simulink library "HDL_ieee_8021513"  (R2024a)
settings: Solver=FixedStepDiscrete  StartTime=0.0  StopTime=10.0  RelTol=1e-3
undefined symbols (not defined in the file or in its folder): Add, axiWidth, channelCyclicPrefixLen, channelDataCarriers, channelEstReference, channelLUT, channelOFDMSamples, channelScramblerInit, decimatorDelay, decimatorFilter, fPHY, frequencyOffsetTimeWindow, fs, headerBitsPerFec, headerBitsPerOFDMSymbol, headerBitsPerSubcarrier, headerCyclicPrefixLen, headerDataCarriers, headerOFDMSamples, headerScramblerInit, interpolatorDelay, interpolatorFilter, leftGuard, N, ncoCarrierFrequency, ncoWordLength, numDataCarriers, oversamplingFactor, payloadBitsPerFec, payloadScramblerInit, payloadWordsPerBlock0, peakDetectorThreshold, peakDetectorWindow, preambleCyclicPrefixLen, preambleDataCarriers, preambleLUT, preambleOFDMSamples, preambleScramblerInit, QAM, rightGuard, Shift
libraries: hdlsllib x198, $bdroot x80, whdlutilities x28, whdledac x10, whdlmod x7, simulink x4, dsphdlfiltering2 x2, dsphdlsigops2 x2, commhdlcrc x2, dspsigops x2, dspstat3 x2, commdigbbndam3 x2
(part 5 of 5)

== system HDL_ieee_8021513/full_tx/store_frame_in_ram/read_frame_from_ram ==
  start_reading : Inport
  ram_size : Inport  Port=2
  bits_per_subcarrier : Inport  Port=3
  cp_len_in : Inport  Port=4
  Enable : EnablePort
  HDL Counter1 : hdlsllib/Sources/HDL Counter  CountType=Free running  CountInit=0  CountStep=1  CountMax=preambleDataCarriers + channelDataCarriers + headerDataCarriers - 1  CountFromType=Initial value  CountFrom=0  CountResetPort=on  CountLoadPort=off  CountEnbPort=on  CountDirPort=off  CountHitOutputPort=off  CountDataType=Unsigned  CountWordLen=16  CountFracLen=0  CountSampTime=1
  Logical Operator5 : Logic  Operator=OR  AllPortsSameDT=off  OutDataTypeStr=boolean
  Relational Operator1 : RelationalOperator  Operator===  OutDataTypeStr=boolean  InputSameDT=off
  State Control : StateControl  StateControl=Synchronous
  Switch1 : Switch  Criteria=u2 ~= 0  SaturateOnIntegerOverflow=off  InputSameDT=off
  Unit Delay1 : UnitDelay  SampleTime=-1  HasFrameUpgradeWarning=on
  bits_selector : Subsystem
  cp_len_creator : Subsystem
  init_selector : Subsystem
  valid_frame : Subsystem
  rd_addr : Outport  VectorParamsAs1DForOutWhenUnconnected=off
  valid_out : Outport  Port=2  VectorParamsAs1DForOutWhenUnconnected=off
  bits_per_subcarrier_out : Outport  Port=3  VectorParamsAs1DForOutWhenUnconnected=off
  init : Outport  Port=4  VectorParamsAs1DForOutWhenUnconnected=off
  new : Outport  Port=5  VectorParamsAs1DForOutWhenUnconnected=off
  cp_len : Outport  Port=6  VectorParamsAs1DForOutWhenUnconnected=off
  wires:
  Switch1/1 -> Unit Delay1/1, valid_frame/1(valid_in), HDL Counter1/2
  bits_selector/1(bits_per_subcarrier_out) -> bits_per_subcarrier_out/1
  Unit Delay1/1 -> Switch1/3
  bits_per_subcarrier/1 -> bits_selector/2(bits_per_subcarrier)
  cp_len_creator/1(cp_len) -> cp_len/1
  init_selector/1(init) -> init/1
  Logical Operator5/1 -> Switch1/2
  cp_len_in/1 -> cp_len_creator/2(cp_len_in)
  Relational Operator1/1 -> Logical Operator5/2
  HDL Counter1/1 -> rd_addr/1, Relational Operator1/2, bits_selector/1(rd_addr), cp_len_creator/1(rd_addr), init_selector/1(rd_addr)  "rd_addr"
  start_reading/1 -> HDL Counter1/1, Logical Operator5/1, Switch1/1
  ram_size/1 -> Relational Operator1/1
  valid_frame/1(valid_out) -> valid_out/1
  valid_frame/2(new) -> new/1

== system HDL_ieee_8021513/full_tx/store_frame_in_ram/write_frame_to_ram ==
  preamble : Inport
  preamble_valid : Inport  Port=2
  channel : Inport  Port=3
  channel_valid : Inport  Port=4
  header : Inport  Port=5
  header_valid : Inport  Port=6
  payload : Inport  Port=7
  payload_valid : Inport  Port=8
  payload_len : Inport  Port=9
  Add1 : Sum
  Constant43 : Constant  Value=numDataCarriers  OutDataTypeStr=uint8  SampleTime=-1
  Constant73 : Constant  Value=preambleDataCarriers + channelDataCarriers + headerDataCarriers - 1  OutDataTypeStr=fixdt(0,13,0)  SampleTime=-1
  Delay3 : Delay  DelayLength=1  InitialCondition=0  UseCircularBuffer=on
  Delay8 : Delay  DelayLength=1  InitialCondition=0  UseCircularBuffer=on
  Delay9 : Delay  DelayLength=1  InitialCondition=1  UseCircularBuffer=on
  HDL Counter : hdlsllib/Sources/HDL Counter  CountType=Free running  CountInit=0  CountStep=1  CountMax=preambleDataCarriers + channelDataCarriers + headerDataCarriers - 1  CountFromType=Initial value  CountFrom=0  CountResetPort=on  CountLoadPort=off  CountEnbPort=on  CountDirPort=off  CountHitOutputPort=off  CountDataType=Unsigned  CountWordLen=16  CountFracLen=0  CountSampTime=1
  Logical Operator : Logic  Operator=OR  Inputs=4  IconShape=distinctive  AllPortsSameDT=off  OutDataTypeStr=boolean
  Product : Product
  Relational Operator : RelationalOperator  Operator===  OutDataTypeStr=boolean  InputSameDT=off
  State Control : StateControl  StateControl=Synchronous
  ram_formatting : Subsystem
  write_data : Outport  VectorParamsAs1DForOutWhenUnconnected=off
  wr_addr : Outport  Port=2  VectorParamsAs1DForOutWhenUnconnected=off
  we : Outport  Port=3  VectorParamsAs1DForOutWhenUnconnected=off
  end : Outport  Port=4  VectorParamsAs1DForOutWhenUnconnected=off
  ram_size : Outport  Port=5  VectorParamsAs1DForOutWhenUnconnected=off
  wires:
  Delay3/1 -> HDL Counter/1, end/1
  channel_valid/1 -> Logical Operator/2, ram_formatting/2(channel_valid)
  header_valid/1 -> Logical Operator/3, ram_formatting/3(header_valid)
  Relational Operator/1 -> Delay3/1
  Logical Operator/1 -> HDL Counter/2, we/1  "we"
  HDL Counter/1 -> Relational Operator/2, wr_addr/1  "wr_addr"
  preamble_valid/1 -> ram_formatting/1(preamble_valid), Logical Operator/1
  payload_valid/1 -> Logical Operator/4, ram_formatting/4(payload_valid)
  preamble/1 -> ram_formatting/5(preamble)
  channel/1 -> ram_formatting/6(channel)
  header/1 -> ram_formatting/7(header)
  payload/1 -> ram_formatting/8(payload)
  ram_formatting/1(Out1) -> write_data/1
  Add1/1 -> Delay9/1
  Constant73/1 -> Add1/1
  Constant43/1 -> Product/1
  payload_len/1 -> Product/2  "payload_len"
  Product/1 -> Delay8/1
  Delay9/1 -> Relational Operator/1, ram_size/1
  Delay8/1 -> Add1/2

== system HDL_ieee_8021513/ofdm_symbol_sync/m_cox/calculate_P ==
  r(d) : Inport
  Add : Sum  OutDataTypeStr=Inherit: Same as first input
  Add1 : Sum  OutDataTypeStr=Inherit: Same as first input
  Complex to Real-Imag : ComplexToRealImag
  Conjugate1 : Math  Operator=conj  SignedPower=on  OutputSignalType=complex  RndMeth=Zero
  Conjugate2 : Math  Operator=conj  SignedPower=on  OutputSignalType=complex  RndMeth=Zero
  Delay{,3..13} (12 alike) : Delay  DelayLength=1  InitialCondition=0  UseCircularBuffer=on
  Delay1 : Delay  DelayLength=(N+preambleCyclicPrefixLen)*5  InitialCondition=0  UseCircularBuffer=on
  Delay2 : Delay  DelayLength=(N+preambleCyclicPrefixLen)*5  InitialCondition=0  UseCircularBuffer=on
  Product{,1..3} (4 alike) : Product  OutDataTypeStr=Inherit: Same as first input
  Subtract1 : Sum  Inputs=+-  OutDataTypeStr=Inherit: Same as first input
  |P(d)|2 : Outport
  P(d) : Outport  Port=2  VectorParamsAs1DForOutWhenUnconnected=off
  wires:
  Delay13/1 -> |P(d)|2/1
  Add1/1 -> Delay13/1
  Delay11/1 -> Add1/2
  Delay12/1 -> Add1/1
  Product3/1 -> Delay12/1
  Product2/1 -> Delay11/1
  Complex to Real-Imag/2 -> Product2/2, Product2/1
  Complex to Real-Imag/1 -> Product3/1, Product3/2
  Conjugate2/1 -> Delay7/1
  Conjugate1/1 -> Delay8/1
  Delay10/1 -> Product1/1
  Delay9/1 -> Product/1
  Delay8/1 -> Product1/2
  Delay7/1 -> Product/2
  Delay6/1 -> Subtract1/1
  Delay5/1 -> Subtract1/2
  Subtract1/1 -> Add/1
  Add/1 -> Delay/1
  Product/1 -> Delay5/1
  Product1/1 -> Delay6/1
  Delay2/1 -> Conjugate2/1  "r(d)"
  Delay1/1 -> Delay2/1, Conjugate1/1, Delay9/1  "r(d+L)"
  r(d)/1 -> Delay1/1, Delay10/1  "r(d+2L)"
  Delay/1 -> Delay3/1, Add/2, Complex to Real-Imag/1  "P(d)"
  Delay3/1 -> Delay4/1
  Delay4/1 -> P(d)/1

== system HDL_ieee_8021513/ofdm_symbol_sync/m_cox/calculate_R ==
  r(d) : Inport
  Add : Sum  OutDataTypeStr=Inherit: Same as first input
  Add1 : Sum  OutDataTypeStr=Inherit: Same as first input
  Complex to Real-Imag : ComplexToRealImag
  Delay : Delay  DelayLength=(N+preambleCyclicPrefixLen)*2*5  InitialCondition=0  UseCircularBuffer=on
  Delay{1..2,4..5,11..12} (6 alike) : Delay  DelayLength=1  InitialCondition=0  UseCircularBuffer=on
  Divide by 2 : hdlsllib/Logic and Bit Operations/Bit Shift  mode=Shift Right Arithmetic  N=1
  Product : Product  OutDataTypeStr=Inherit: Same as first input
  Product1 : Product  OutDataTypeStr=Inherit: Same as first input
  Product2 : Product  OutDataTypeStr=Inherit: Same as first input
  Subtract : Sum  Inputs=+-  OutDataTypeStr=Inherit: Same as first input
  Rf2 : Outport
  wires:
  Complex to Real-Imag/2 -> Product/2, Product/1
  Product/1 -> Delay11/1
  Add1/1 -> Delay4/1
  r(d)/1 -> Complex to Real-Imag/1  "P(d)"
  Delay11/1 -> Add1/2
  Complex to Real-Imag/1 -> Product1/1, Product1/2
  Delay12/1 -> Add1/1
  Delay5/1 -> Product2/2, Product2/1
  Delay4/1 -> Delay/1, Subtract/1  "|r(d+2L)|2"
  Delay2/1 -> Rf2/1
  Subtract/1 -> Add/1
  Add/1 -> Delay1/1
  Divide by 2/1 -> Delay5/1
  Delay1/1 -> Divide by 2/1, Add/2
  Delay/1 -> Subtract/2  "|r(d)|2"
  Product1/1 -> Delay12/1
  Product2/1 -> Delay2/1

== system HDL_ieee_8021513/full_tx/store_frame_in_ram/read_frame_from_ram/bits_selector ==
  rd_addr : Inport
  bits_per_subcarrier : Inport  Port=2
  Compare To Constant : hdlsllib/Logic and Bit Operations/Compare To Constant  relop=<=  const=preambleDataCarriers-1  OutDataTypeStr=boolean
  Compare To Constant1 : hdlsllib/Logic and Bit Operations/Compare To Constant  relop=<=  const=preambleDataCarriers + channelDataCarriers -1  OutDataTypeStr=boolean
  Compare To Constant2 : hdlsllib/Logic and Bit Operations/Compare To Constant  relop=<=  const=preambleDataCarriers + channelDataCarriers + headerDataCarriers-1  OutDataTypeStr=boolean
  Constant : Constant  OutDataTypeStr=fixdt(0,4,0)  SampleTime=-1
  Constant1 : Constant  OutDataTypeStr=fixdt(0,4,0)  SampleTime=-1
  Constant2 : Constant  Value=2  OutDataTypeStr=fixdt(0,4,0)  SampleTime=-1
  Delay : Delay  DelayLength=1  InitialCondition=0  UseCircularBuffer=on
  Multiport Switch : MultiPortSwitch  DataPortOrder=Zero-based contiguous  Inputs=4  zeroidx=on  SaturateOnIntegerOverflow=off  InputSameDT=off
  one_hot_coder : Subsystem
  bits_per_subcarrier_out : Outport
  wires:
  Compare To Constant1/1 -> one_hot_coder/2(channel)
  one_hot_coder/1(bits_per_subcarrier_select) -> Delay/1
  Compare To Constant/1 -> one_hot_coder/1(preamble)
  Constant2/1 -> Multiport Switch/4
  Constant1/1 -> Multiport Switch/3
  Constant/1 -> Multiport Switch/2
  Compare To Constant2/1 -> one_hot_coder/3(header)
  rd_addr/1 -> Compare To Constant2/1, Compare To Constant/1, Compare To Constant1/1
  Multiport Switch/1 -> bits_per_subcarrier_out/1
  Delay/1 -> Multiport Switch/1
  bits_per_subcarrier/1 -> Multiport Switch/5

== system HDL_ieee_8021513/full_tx/store_frame_in_ram/read_frame_from_ram/cp_len_creator ==
  rd_addr : Inport
  cp_len_in : Inport  Port=2
  Bits to Word : hdlsllib/Logic and Bit Operations/Bits to Word
  Compare To Constant : hdlsllib/Logic and Bit Operations/Compare To Constant  relop=<=  const=preambleDataCarriers-1  OutDataTypeStr=boolean
  Compare To Constant1 : hdlsllib/Logic and Bit Operations/Compare To Constant  relop=<=  const=preambleDataCarriers + channelDataCarriers -1  OutDataTypeStr=boolean
  Compare To Constant2 : hdlsllib/Logic and Bit Operations/Compare To Constant  relop=<=  const=preambleDataCarriers + channelDataCarriers + headerDataCarriers-1  OutDataTypeStr=boolean
  Constant : Constant  Value=preambleCyclicPrefixLen  OutDataTypeStr=uint8  SampleTime=-1
  Constant1 : Constant  Value=channelCyclicPrefixLen  OutDataTypeStr=uint8  SampleTime=-1
  Constant2 : Constant  Value=headerCyclicPrefixLen  OutDataTypeStr=uint8  SampleTime=-1
  Constant3 : Constant  Value=N/32  OutDataTypeStr=fixdt(0,4,0)  SampleTime=-1
  Data Type Conversion : DataTypeConversion  OutDataTypeStr=fixdt(0,1,0)  SaturateOnIntegerOverflow=off  RndMeth=Floor
  Delay : Delay  DelayLength=1  InitialCondition=0  UseCircularBuffer=on
  Delay1 : Delay  DelayLength=1  InitialCondition=0  UseCircularBuffer=on
  Multiport Switch : MultiPortSwitch  DataPortOrder=Zero-based contiguous  Inputs=4  zeroidx=on  OutDataTypeStr=uint8  SaturateOnIntegerOverflow=off
  Product : Product  OutDataTypeStr=uint8
  one_hot_coder : Subsystem
  cp_len : Outport
  wires:
  rd_addr/1 -> Compare To Constant2/1, Compare To Constant/1, Compare To Constant1/1
  Compare To Constant/1 -> one_hot_coder/1(preamble)
  Compare To Constant1/1 -> one_hot_coder/2(channel)
  Compare To Constant2/1 -> one_hot_coder/3(header)
  Constant/1 -> Multiport Switch/2
  Constant1/1 -> Multiport Switch/3
  Constant2/1 -> Multiport Switch/4
  Multiport Switch/1 -> cp_len/1
  one_hot_coder/1(cp_select) -> Delay/1
  Delay/1 -> Multiport Switch/1
  Constant3/1 -> Product/1
  cp_len_in/1 -> Data Type Conversion/1
  Product/1 -> Delay1/1
  Data Type Conversion/1 -> Bits to Word/1
  Bits to Word/1 -> Product/2
  Delay1/1 -> Multiport Switch/5

== system HDL_ieee_8021513/full_tx/store_frame_in_ram/read_frame_from_ram/init_selector ==
  rd_addr : Inport
  Compare To Constant : hdlsllib/Logic and Bit Operations/Compare To Constant  relop=<=  const=preambleDataCarriers-1  OutDataTypeStr=boolean
  Compare To Constant1 : hdlsllib/Logic and Bit Operations/Compare To Constant  relop=<=  const=preambleDataCarriers + channelDataCarriers -1  OutDataTypeStr=boolean
  Compare To Constant2 : hdlsllib/Logic and Bit Operations/Compare To Constant  relop=<=  const=preambleDataCarriers + channelDataCarriers + headerDataCarriers-1  OutDataTypeStr=boolean
  Constant : Constant  Value=preambleScramblerInit  OutDataTypeStr=boolean  SampleTime=-1
  Constant1 : Constant  Value=channelScramblerInit  OutDataTypeStr=boolean  SampleTime=-1
  Constant2 : Constant  Value=headerScramblerInit  OutDataTypeStr=boolean  SampleTime=-1
  Constant3 : Constant  Value=payloadScramblerInit  OutDataTypeStr=boolean  SampleTime=-1
  Delay : Delay  DelayLength=1  InitialCondition=0  UseCircularBuffer=on
  Multiport Switch : MultiPortSwitch  DataPortOrder=Zero-based contiguous  Inputs=4  zeroidx=on  SaturateOnIntegerOverflow=off  InputSameDT=off
  one_hot_coder : Subsystem
  init : Outport
  wires:
  Compare To Constant1/1 -> one_hot_coder/2(channel)
  one_hot_coder/1(cp_select) -> Delay/1
  Compare To Constant/1 -> one_hot_coder/1(preamble)
  Constant2/1 -> Multiport Switch/4
  Constant1/1 -> Multiport Switch/3
  Constant/1 -> Multiport Switch/2
  Compare To Constant2/1 -> one_hot_coder/3(header)
  rd_addr/1 -> Compare To Constant2/1, Compare To Constant/1, Compare To Constant1/1
  Multiport Switch/1 -> init/1
  Delay/1 -> Multiport Switch/1
  Constant3/1 -> Multiport Switch/5

== system HDL_ieee_8021513/full_tx/store_frame_in_ram/read_frame_from_ram/valid_frame ==
  valid_in : Inport
  Compare To Zero1 : hdlsllib/Logic and Bit Operations/Compare To Zero  relop===  OutDataTypeStr=boolean
  Delay4 : Delay  InitialCondition=0  UseCircularBuffer=on
  HDL Counter2 : hdlsllib/Sources/HDL Counter  CountType=Count limited  CountInit=0  CountStep=1  CountMax=numDataCarriers-1  CountFromType=Initial value  CountFrom=0  CountResetPort=off  CountLoadPort=off  CountEnbPort=on  CountDirPort=off  CountHitOutputPort=off  CountDataType=Unsigned  CountWordLen=nextpow2(numDataCarriers)  CountFracLen=0  CountSampTime=1
  Logical Operator4 : Logic  IconShape=distinctive  AllPortsSameDT=off  OutDataTypeStr=boolean
  valid_out : Outport  VectorParamsAs1DForOutWhenUnconnected=off
  new : Outport  Port=2  VectorParamsAs1DForOutWhenUnconnected=off
  wires:
  Logical Operator4/1 -> new/1
  Delay4/1 -> valid_out/1, Logical Operator4/1, HDL Counter2/1
  HDL Counter2/1 -> Compare To Zero1/1
  valid_in/1 -> Delay4/1
  Compare To Zero1/1 -> Logical Operator4/2

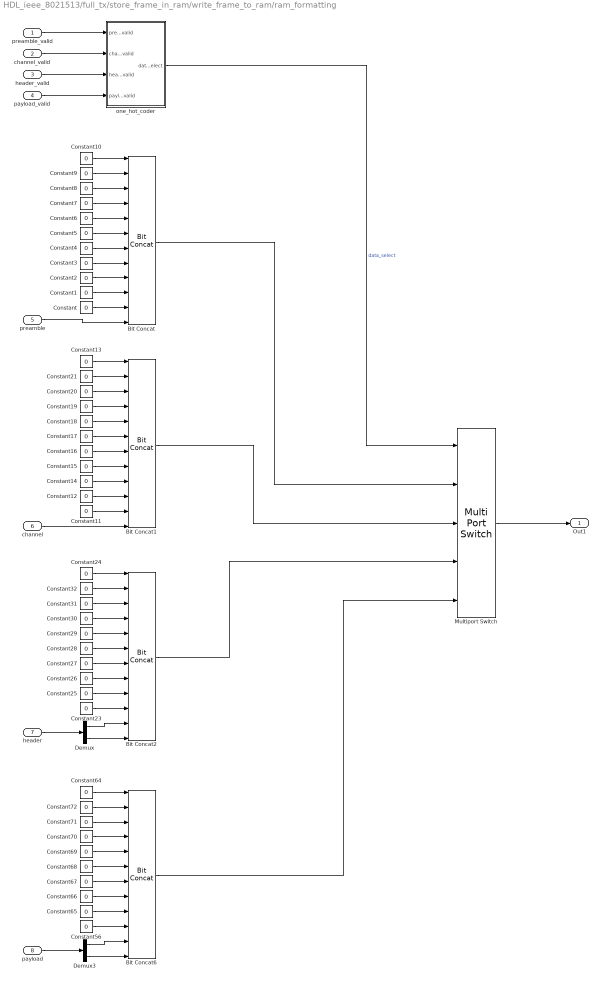
== system HDL_ieee_8021513/full_tx/store_frame_in_ram/write_frame_to_ram/ram_formatting ==
  preamble_valid : Inport
  channel_valid : Inport  Port=2
  header_valid : Inport  Port=3
  payload_valid : Inport  Port=4
  preamble : Inport  Port=5
  channel : Inport  Port=6
  header : Inport  Port=7
  payload : Inport  Port=8
  Bit Concat{,1..2,6} (4 alike) : hdlsllib/Logic and Bit Operations/Bit Concat  numInputs=12
  Constant{,1..21,23..32,56,64..72} (42 alike) : Constant  Value=0  OutDataTypeStr=boolean  SampleTime=-1
  Demux : Demux  Outputs=2
  Demux3 : Demux  Outputs=2
  Multiport Switch : MultiPortSwitch  DataPortOrder=Zero-based contiguous  Inputs=4  zeroidx=on  SaturateOnIntegerOverflow=off  InputSameDT=off
  one_hot_coder : Subsystem
  Out1 : Outport
  wires:
  channel/1 -> Bit Concat1/12
  Constant32/1 -> Bit Concat2/2
  Constant68/1 -> Bit Concat6/6
  Constant23/1 -> Bit Concat2/10
  Constant29/1 -> Bit Concat2/5
  Constant31/1 -> Bit Concat2/3
  Constant3/1 -> Bit Concat/8
  Constant24/1 -> Bit Concat2/1
  Constant12/1 -> Bit Concat1/10
  header_valid/1 -> one_hot_coder/3(header_valid)
  Bit Concat1/1 -> Multiport Switch/3
  Constant4/1 -> Bit Concat/7
  Constant13/1 -> Bit Concat1/1
  Constant64/1 -> Bit Concat6/1
  Constant14/1 -> Bit Concat1/9
  Constant18/1 -> Bit Concat1/5
  Constant71/1 -> Bit Concat6/3
  Constant56/1 -> Bit Concat6/10
  Constant67/1 -> Bit Concat6/7
  Constant6/1 -> Bit Concat/5
  Constant65/1 -> Bit Concat6/9
  Constant20/1 -> Bit Concat1/3
  Bit Concat2/1 -> Multiport Switch/4
  Constant30/1 -> Bit Concat2/4
  header/1 -> Demux/1
  payload/1 -> Demux3/1
  Constant17/1 -> Bit Concat1/6
  Demux/2 -> Bit Concat2/12
  Constant27/1 -> Bit Concat2/7
  Constant16/1 -> Bit Concat1/7
  Constant72/1 -> Bit Concat6/2
  Constant69/1 -> Bit Concat6/5
  Constant/1 -> Bit Concat/11
  Constant11/1 -> Bit Concat1/11
  Constant25/1 -> Bit Concat2/9
  Constant70/1 -> Bit Concat6/4
  one_hot_coder/1(data_select) -> Multiport Switch/1  "data_select"
  Constant19/1 -> Bit Concat1/4
  Constant21/1 -> Bit Concat1/2
  Constant1/1 -> Bit Concat/10
  Bit Concat6/1 -> Multiport Switch/5
  preamble/1 -> Bit Concat/12
  channel_valid/1 -> one_hot_coder/2(channel_valid)
  Constant10/1 -> Bit Concat/1
  Constant28/1 -> Bit Concat2/6
  Demux3/2 -> Bit Concat6/12
  preamble_valid/1 -> one_hot_coder/1(preamble_valid)
  Constant5/1 -> Bit Concat/6
  Constant15/1 -> Bit Concat1/8
  Constant66/1 -> Bit Concat6/8
  Multiport Switch/1 -> Out1/1
  payload_valid/1 -> one_hot_coder/4(payload_valid)
  Constant9/1 -> Bit Concat/2
  Demux/1 -> Bit Concat2/11
  Demux3/1 -> Bit Concat6/11
  Constant2/1 -> Bit Concat/9
  Constant7/1 -> Bit Concat/4
  Bit Concat/1 -> Multiport Switch/2
  Constant8/1 -> Bit Concat/3
  Constant26/1 -> Bit Concat2/8

== system HDL_ieee_8021513/full_tx/store_frame_in_ram/read_frame_from_ram/bits_selector/one_hot_coder ==
  preamble : Inport
  channel : Inport  Port=2
  header : Inport  Port=3
  Bit Concat : hdlsllib/Logic and Bit Operations/Bit Concat  numInputs=2
  Logical Operator : Logic  Operator=NOT  IconShape=distinctive  AllPortsSameDT=off  OutDataTypeStr=boolean
  Logical Operator1 : Logic  IconShape=distinctive  AllPortsSameDT=off  OutDataTypeStr=boolean
  Logical Operator2 : Logic  Operator=OR  IconShape=distinctive  AllPortsSameDT=off  OutDataTypeStr=boolean
  Logical Operator3 : Logic  Operator=NOT  IconShape=distinctive  AllPortsSameDT=off  OutDataTypeStr=boolean
  Logical Operator4 : Logic  Operator=NOT  IconShape=distinctive  AllPortsSameDT=off  OutDataTypeStr=boolean
  bits_per_subcarrier_select : Outport
  wires:
  Bit Concat/1 -> bits_per_subcarrier_select/1
  channel/1 -> Logical Operator1/2, Logical Operator/1
  preamble/1 -> Logical Operator3/1
  Logical Operator3/1 -> Logical Operator1/1
  header/1 -> Logical Operator4/1
  Logical Operator1/1 -> Logical Operator2/1
  Logical Operator4/1 -> Logical Operator2/2
  Logical Operator/1 -> Bit Concat/1
  Logical Operator2/1 -> Bit Concat/2

== system HDL_ieee_8021513/full_tx/store_frame_in_ram/read_frame_from_ram/cp_len_creator/one_hot_coder ==
  preamble : Inport
  channel : Inport  Port=2
  header : Inport  Port=3
  Bit Concat : hdlsllib/Logic and Bit Operations/Bit Concat  numInputs=2
  Logical Operator : Logic  Operator=NOT  IconShape=distinctive  AllPortsSameDT=off  OutDataTypeStr=boolean
  Logical Operator1 : Logic  IconShape=distinctive  AllPortsSameDT=off  OutDataTypeStr=boolean
  Logical Operator2 : Logic  Operator=OR  IconShape=distinctive  AllPortsSameDT=off  OutDataTypeStr=boolean
  Logical Operator3 : Logic  Operator=NOT  IconShape=distinctive  AllPortsSameDT=off  OutDataTypeStr=boolean
  Logical Operator4 : Logic  Operator=NOT  IconShape=distinctive  AllPortsSameDT=off  OutDataTypeStr=boolean
  cp_select : Outport
  wires:
  channel/1 -> Logical Operator1/2, Logical Operator/1
  Logical Operator/1 -> Bit Concat/1
  preamble/1 -> Logical Operator3/1
  Logical Operator3/1 -> Logical Operator1/1
  header/1 -> Logical Operator4/1
  Logical Operator1/1 -> Logical Operator2/1
  Logical Operator2/1 -> Bit Concat/2
  Logical Operator4/1 -> Logical Operator2/2
  Bit Concat/1 -> cp_select/1

== system HDL_ieee_8021513/full_tx/store_frame_in_ram/read_frame_from_ram/init_selector/one_hot_coder ==
  preamble : Inport
  channel : Inport  Port=2
  header : Inport  Port=3
  Bit Concat : hdlsllib/Logic and Bit Operations/Bit Concat  numInputs=2
  Logical Operator : Logic  Operator=NOT  IconShape=distinctive  AllPortsSameDT=off  OutDataTypeStr=boolean
  Logical Operator1 : Logic  IconShape=distinctive  AllPortsSameDT=off  OutDataTypeStr=boolean
  Logical Operator2 : Logic  Operator=OR  IconShape=distinctive  AllPortsSameDT=off  OutDataTypeStr=boolean
  Logical Operator3 : Logic  Operator=NOT  IconShape=distinctive  AllPortsSameDT=off  OutDataTypeStr=boolean
  Logical Operator4 : Logic  Operator=NOT  IconShape=distinctive  AllPortsSameDT=off  OutDataTypeStr=boolean
  cp_select : Outport
  wires:
  Bit Concat/1 -> cp_select/1
  channel/1 -> Logical Operator1/2, Logical Operator/1
  preamble/1 -> Logical Operator3/1
  Logical Operator3/1 -> Logical Operator1/1
  header/1 -> Logical Operator4/1
  Logical Operator1/1 -> Logical Operator2/1
  Logical Operator4/1 -> Logical Operator2/2
  Logical Operator/1 -> Bit Concat/1
  Logical Operator2/1 -> Bit Concat/2

== system HDL_ieee_8021513/full_tx/store_frame_in_ram/write_frame_to_ram/ram_formatting/one_hot_coder ==
  preamble_valid : Inport
  channel_valid : Inport  Port=2
  header_valid : Inport  Port=3
  payload_valid : Inport  Port=4
  Bit Concat : hdlsllib/Logic and Bit Operations/Bit Concat  numInputs=2
  Logical Operator : Logic  Operator=OR  IconShape=distinctive  AllPortsSameDT=off  OutDataTypeStr=boolean
  Logical Operator1 : Logic  Operator=OR  IconShape=distinctive  AllPortsSameDT=off  OutDataTypeStr=boolean
  Terminator : Terminator
  data_select : Outport
  wires:
  Bit Concat/1 -> data_select/1
  header_valid/1 -> Logical Operator/1
  channel_valid/1 -> Logical Operator1/2
  payload_valid/1 -> Logical Operator/2, Logical Operator1/1
  preamble_valid/1 -> Terminator/1
  Logical Operator1/1 -> Bit Concat/2
  Logical Operator/1 -> Bit Concat/1
